simulink model "gcs"  (R2014b)
settings: Solver=ode45  StartTime=0.0  StopTime=100  RelTol=1e-3
libraries: rtwinlib x1, dspnetwork x1
settings Model: Creator=Magnus Blomberg  LastModifiedBy=Magnus Blomberg

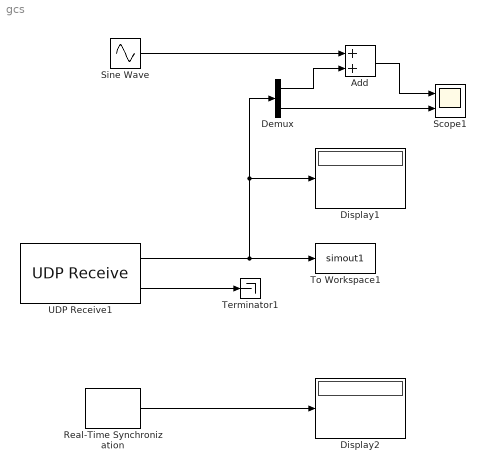
== system gcs ==
  Add : Sum
  Demux : Demux  Outputs=2
  Display1 : Display
  Display2 : Display
  Real-Time Synchronization : rtwinlib/Real-Time Synchronization  SampleTime=0.2  MaxMissedTicks=100  ShowMissedTicks=on  YieldWhenWaiting=off
  Scope1 : Scope  NumInputPorts=2
      settings: TickLabels=on  ShowLegends=on  TimeRange=100  YMin=-100~-1  YMax=100~1  ScrollMode=on
  Sine Wave : Sin  Amplitude=0  SampleTime=0
  Terminator1 : Terminator
  To Workspace1 : ToWorkspace  VariableName=simout1  SaveFormat=Timeseries  SampleTime=-1
  UDP Receive1 : dspnetwork/UDP Receive  localURL='0.0.0.0'  localPort=27001  remoteURL='0.0.0.0'  remotePort=-1  recvBufferSize=1000  dims=3  signalDatatype=double  isVarSize=off  showBlockingTime=on  blockingTime=0  sampletime=.02  blockPlatform=BeagleBone
  wires:
  UDP Receive1/2 -> Terminator1/1
  UDP Receive1/1 -> To Workspace1/1, Display1/1, Demux/1
  Sine Wave/1 -> Add/1
  Demux/1 -> Add/2
  Add/1 -> Scope1/1
  Demux/2 -> Scope1/2
  Real-Time Synchronization/1 -> Display2/1
